simulink model "M9_ex3"  (R2022a)
settings: Solver=VariableStepAuto  StartTime=0.0  StopTime=1000  RelTol=1e-3
libraries: slpidlib x1
settings Model: Creator=hntran  LastModifiedBy=hntran

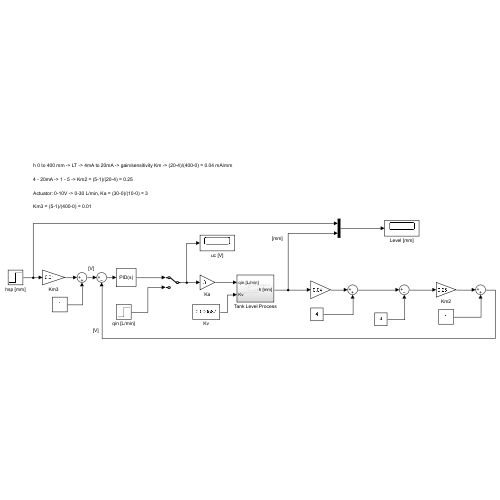
[thumbnail: Simulink's stored preview of the top-level diagram]
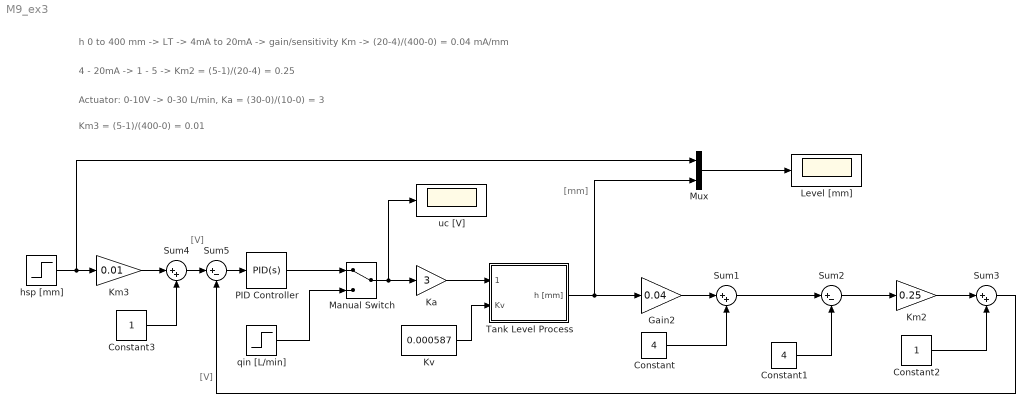
== system M9_ex3 ==
  note: [V]
  note: [V]
  note: Km3 = (5-1)/(400-0) = 0.01
  note: Actuator: 0-10V -> 0-30 L/min, Ka = (30-0)/(10-0) = 3
  note: [mm]
  note: h 0 to 400 mm -> LT -> 4mA to 20mA -> gain/sensitivity Km -> (20-4)/(400-0) = 0.04 mA/mm
  note: 4 - 20mA -> 1 - 5 -> Km2 = (5-1)/(20-4) = 0.25
  Constant : Constant  Value=4
  Constant1 : Constant  Value=4
  Constant2 : Constant
  Constant3 : Constant
  Gain2 : Gain  Gain=0.04
  Ka : Gain  Gain=3
  Km2 : Gain  Gain=0.25
  Km3 : Gain  Gain=0.01
  Kv : Constant  Value=0.000587
  Level [mm] : Scope
  Manual Switch : ManualSwitch
  Mux : Mux  Inputs=2
  PID Controller : slpidlib/PID Controller  Controller=PID  Form=Parallel  TimeDomain=Continuous-time  UseExternalTs=off  SampleTime=-1  IntegratorMethod=Forward Euler  FilterMethod=Forward Euler  ControllerParametersSource=internal  P=2.5  I=0.125  UseKiTs=off  D=0.25  N=100  UseFilter=on  TunerSelectOption=Transfer Function Based (PID Tuner App)  InitialConditionSource=internal  InitialConditionForIntegrator=0  InitialConditionForFilter=0  DifferentiatorICPrevScaledInput=0  ExternalReset=none  TrackingMode=off  Kt=1  LimitOutput=off  SatLimitsSource=internal  UpperSaturationLimit=inf  LowerSaturationLimit=-inf  LinearizeAsGain=on  AntiWindupMode=none  Kb=1  POutMin=[]  POutMax=[]  IOutMin=[]  IOutMax=[]  DOutMin=[]  DOutMax=[]  NOutMin=[]  NOutMax=[]  SumOutMin=[]  SumOutMax=[]  SaturationOutMin=[]  SaturationOutMax=[]  PParamMin=[]  PParamMax=[]  IParamMin=[]  IParamMax=[]  DParamMin=[]  DParamMax=[]  NParamMin=[]  NParamMax=[]  KbParamMin=[]  KbParamMax=[]  KtParamMin=[]  KtParamMax=[]  KbOutMin=[]  KbOutMax=[]  KtOutMin=[]  KtOutMax=[]  IntegratorOutMin=[]  IntegratorOutMax=[]  FilterOutMin=[]  FilterOutMax=[]  SumI1OutMin=[]  SumI1OutMax=[]  SumI2OutMin=[]  SumI2OutMax=[]  SumI3OutMin=[]  SumI3OutMax=[]  SumI4OutMin=[]  SumI4OutMax=[]  SumDOutMin=[]  SumDOutMax=[]  DifferentiatorOutMin=[]  DifferentiatorOutMax=[]  FilterDiffOutCoefMin=[]  FilterDiffOutCoefMax=[]  ReciprocalOutMin=[]  ReciprocalOutMax=[]  SumDenOutMin=[]  SumDenOutMax=[]  SumNumOutMin=[]  SumNumOutMax=[]  DivideOutMin=[]  DivideOutMax=[]  UdiffTsProdOutMin=[]  UdiffTsProdOutMax=[]  NTsProdOutMin=[]  NTsProdOutMax=[]  UintegralTsProdOutMin=[]  UintegralTsProdOutMax=[]  UngainTsProdOutMin=[]  UngainTsProdOutMax=[]  IntegratorContinuousStateAttributes=''  IntegratorStateMustResolveToSignalObject=off  IntegratorRTWStateStorageClass=Auto  FilterContinuousStateAttributes=''  FilterStateMustResolveToSignalObject=off  FilterRTWStateStorageClass=Auto  ParallelPVariant=InternalParameters  IdealPVariant=Disabled  IVariant=InternalParameters  DVariant=InternalParameters  IntegratorVariant=Continuous  SatVariant=Disabled  AWVariant=Passthrough  PCopyVariant=Disabled  TRVariant=Disabled  FdbkBlocksVariant=Forward  IdealPFdbkVariant=Disabled  SatFdbkVariant=Disabled  DerivativeFilterVariant=ContFilter  NVariant=InternalParameters  NCopyVariant=Disabled  FilterICVariant=InternalICsFilter  IntegratorICVariant=InternalICs  ExternalResetVariant=Disabled  TRSumVariant=Passthrough  SumFdbkVariant=Disabled  SumVariant=Sum_PID  TsampFilterVariant=InternalTs  TsampNgainVariant=Passthrough  TsampIntegralVariant=Passthrough  ExternalSaturationOutDataTypeStr=Inherit: Same as second input  aMode=0
  Sum1 : Sum  Inputs=|++
  Sum2 : Sum  Inputs=|+-
  Sum3 : Sum  Inputs=|++
  Sum4 : Sum  Inputs=|++
  Sum5 : Sum  Inputs=|+-
  Tank Level Process : Subsystem
  hsp [mm] : Step  Time=0  After=200  SampleTime=0  ZeroCross=off
  qin [L/min] : Step  Time=0  After=5  SampleTime=0
  uc [V] : Scope
  wires:
  Tank Level Process/1(h [mm]) -> Mux/2, Gain2/1
  Kv/1 -> Tank Level Process/2(Kv)
  Sum1/1 -> Sum2/1
  Constant/1 -> Sum1/2
  Gain2/1 -> Sum1/1
  Constant1/1 -> Sum2/2
  Sum2/1 -> Km2/1
  Km2/1 -> Sum3/1
  Constant2/1 -> Sum3/2
  Ka/1 -> Tank Level Process/1(qin [L/min])
  Manual Switch/1 -> uc [V]/1, Ka/1
  qin [L/min]/1 -> Manual Switch/2
  PID Controller/1 -> Manual Switch/1
  Km3/1 -> Sum4/1
  Constant3/1 -> Sum4/2
  Sum4/1 -> Sum5/1
  Sum5/1 -> PID Controller/1
  Sum3/1 -> Sum5/2
  hsp [mm]/1 -> Mux/1, Km3/1
  Mux/1 -> Level [mm]/1

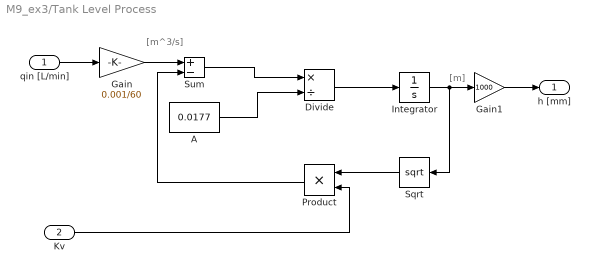
== system M9_ex3/Tank Level Process ==
  note: [m]
  note: [m^3/s]
  qin [L/min] : Inport
  Kv : Inport  Port=2
  A : Constant  Value=0.0177
  Divide : Product  Inputs=*/
  Gain : Gain  Gain=0.001/60
  Gain1 : Gain  Gain=1000
  Integrator : Integrator
  Product : Product
  Sqrt : Sqrt
  Sum : Sum  Inputs=+-
  h [mm] : Outport
  wires:
  Kv/1 -> Product/2
  Sqrt/1 -> Product/1
  Divide/1 -> Integrator/1
  Gain/1 -> Sum/1
  A/1 -> Divide/2
  Integrator/1 -> Gain1/1, Sqrt/1
  Product/1 -> Sum/2
  Sum/1 -> Divide/1
  qin [L/min]/1 -> Gain/1
  Gain1/1 -> h [mm]/1
